simulink model "datarun_final"  (R2018a)
settings: Solver=VariableStepAuto  StartTime=0.0  StopTime=max(all_wheel_out_data(1,:))  RelTol=1e-3
PreLoadFcn:
  | load('all_wheel_out_data.mat');
  | load('bGbAtheta.mat');
  | load('pivot_offs_sws.mat');
  | load('ropod_kinmodel_pv.mat');
  | load('simple_bias_imu.mat');
  | load('simple_bias_gyro.mat');
values from neighbouring files (symbols this model uses):
  pivot_offs_sws = 1*[3.835 3.465 2.059 0.357]    [init_model.m]    (also in pivot_offs_sws.mat = [6.2589 0.5402 0.0584 0.0203])
  ropod_kinmodel_pv = [0.0525 0.0525 0.0525 0.0525 0.0525 0.0525 0.0525 0.0525 0.01 0.08 0.21 0.21 ... (18 elements, 1x18)]    [ropod_kinmodel_pv.mat]    (also in set_ropod_KinModparams.m = struct2array(ropod_kinmodel_param))
  simple_bias_gyro = [bias_gx; bias_gy; bias_gz]    [bias_simple.m]
  simple_bias_imu = [bias_x; bias_y]    [bias_simple.m]
undefined symbols (not defined in the file or in its folder): DiscIntNeverNeededParam
libraries: dspfdesign x12, simulink x5
settings Model: Creator=s151900  LastModifiedBy=s151900

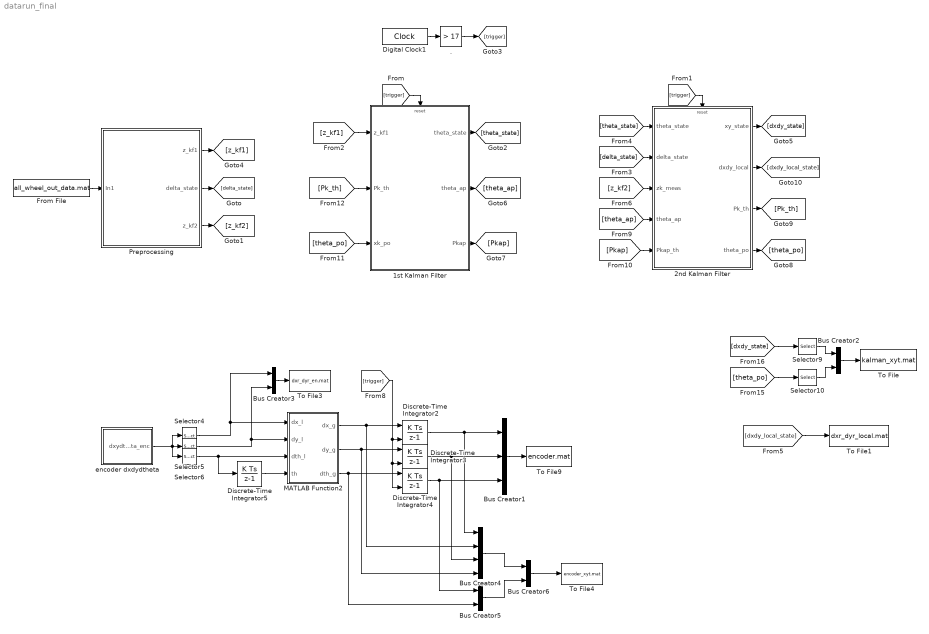
== system datarun_final ==
  . : simulink/Logic and Bit Operations/Compare To Constant  relop=>  const=17  OutDataTypeStr=boolean
  1st Kalman Filter : Subsystem  TreatAsAtomicUnit=on
  2nd Kalman Filter : Subsystem  TreatAsAtomicUnit=on
  Bus Creator1 : BusCreator  Inputs=3
  Bus Creator{2..3,5..6} (4 alike) : BusCreator  Inputs=2
  Bus Creator4 : BusCreator  Inputs=4
  Digital Clock1 : DigitalClock  SampleTime=0.001
  Discrete-Time Integrator2 : DiscreteIntegrator  gainval=1  ExternalReset=rising  SampleTime=-1  ICPrevOutput=DiscIntNeverNeededParam  ICPrevScaledInput=DiscIntNeverNeededParam
  Discrete-Time Integrator3 : DiscreteIntegrator  gainval=1  ExternalReset=rising  SampleTime=-1  ICPrevOutput=DiscIntNeverNeededParam  ICPrevScaledInput=DiscIntNeverNeededParam
  Discrete-Time Integrator4 : DiscreteIntegrator  gainval=1  ExternalReset=rising  InitialCondition=deg2rad(10)  SampleTime=-1  ICPrevOutput=DiscIntNeverNeededParam  ICPrevScaledInput=DiscIntNeverNeededParam
  Discrete-Time Integrator5 : DiscreteIntegrator  gainval=1  InitialCondition=deg2rad(10)  SampleTime=-1  ICPrevOutput=DiscIntNeverNeededParam  ICPrevScaledInput=DiscIntNeverNeededParam
  From File : FromFile  FileName=all_wheel_out_data.mat  SampleTime=0.001
  MATLAB Function2 : MATLAB Function  TreatAsAtomicUnit=on
  Preprocessing : Subsystem
  Selector10 : Selector  InputPortWidth=3  IndexOptions=Index vector (dialog)  Indices=[1 2]  OutputSizes=1
  Selector4 : Selector  InputPortWidth=3  IndexOptions=Index vector (dialog)  Indices=1  OutputSizes=1
  Selector5 : Selector  InputPortWidth=3  IndexOptions=Index vector (dialog)  Indices=2  OutputSizes=1
  Selector6 : Selector  InputPortWidth=3  IndexOptions=Index vector (dialog)  Indices=3  OutputSizes=1
  Selector9 : Selector  InputPortWidth=6  IndexOptions=Index vector (dialog)  Indices=[1 2 4 5]  OutputSizes=1
  To File : ToFile  Filename=kalman_xyt.mat  MatrixName=kalman_xyt
  To File1 : ToFile  Filename=dxr_dyr_local.mat  MatrixName=dxr_dyr_local
  To File3 : ToFile  Filename=dxr_dyr_en.mat  MatrixName=dxr_dyr_en
  To File4 : ToFile  Filename=encoder_xyt.mat  MatrixName=encoder_xyt
  To File9 : ToFile  Filename=encoder.mat
  encoder dxdydtheta : Subsystem
  wires:
  Digital Clock1/1 -> ./1
  From File/1 -> Preprocessing/1(In1)
  1st Kalman Filter/1(theta_state) -> [theta_state]
  Preprocessing/2(delta_state) -> [delta_state]
  Preprocessing/3(z_kf2) -> [z_kf2]
  [theta_state] -> 2nd Kalman Filter/1(theta_state)
  [delta_state] -> 2nd Kalman Filter/2(delta_state)
  [z_kf2] -> 2nd Kalman Filter/3(zk_meas)
  ./1 -> [trigger]
  [trigger] -> 1st Kalman Filter/Reset
  [trigger] -> 2nd Kalman Filter/Reset
  Preprocessing/1(z_kf1) -> [z_kf1]
  [z_kf1] -> 1st Kalman Filter/1(z_kf1)
  2nd Kalman Filter/1(xy_state) -> [dxdy_state]
  Bus Creator1/1 -> To File9/1
  Discrete-Time Integrator2/1 -> Bus Creator4/1, Bus Creator1/1
  Discrete-Time Integrator3/1 -> Bus Creator4/3, Bus Creator1/2
  Discrete-Time Integrator4/1 -> Bus Creator5/1, Bus Creator1/3
  1st Kalman Filter/2(theta_ap) -> [theta_ap]
  1st Kalman Filter/3("Pkap ") -> [Pkap]
  [theta_ap] -> 2nd Kalman Filter/4(theta_ap)
  [Pkap] -> 2nd Kalman Filter/5(Pkap_th)
  [theta_po] -> 1st Kalman Filter/3(xk_po)
  2nd Kalman Filter/4(theta_po) -> [theta_po]
  2nd Kalman Filter/3(Pk_th) -> [Pk_th]
  [Pk_th] -> 1st Kalman Filter/2(Pk_th)
  [theta_po] -> Selector10/1
  Bus Creator2/1 -> To File/1
  [dxdy_state] -> Selector9/1
  Selector10/1 -> Bus Creator2/2
  Selector9/1 -> Bus Creator2/1
  2nd Kalman Filter/2(dxdy_local) -> [dxdy_local_state]
  [dxdy_local_state] -> To File1/1
  Selector6/1 -> Discrete-Time Integrator5/1, MATLAB Function2/3(dth_l)
  Selector5/1 -> Bus Creator3/2, MATLAB Function2/2(dy_l)
  Bus Creator4/1 -> Bus Creator6/1
  encoder dxdydtheta/1(dxydtheta_enc) -> Selector4/1, Selector6/1, Selector5/1
  Bus Creator5/1 -> Bus Creator6/2
  MATLAB Function2/1(dx_g) -> Bus Creator4/2, Discrete-Time Integrator2/1
  Bus Creator3/1 -> To File3/1
  Selector4/1 -> Bus Creator3/1, MATLAB Function2/1(dx_l)
  Bus Creator6/1 -> To File4/1
  Discrete-Time Integrator5/1 -> MATLAB Function2/4(th)
  MATLAB Function2/2(dy_g) -> Discrete-Time Integrator3/1, Bus Creator4/4
  [trigger] -> Discrete-Time Integrator2/2, Discrete-Time Integrator4/2, Discrete-Time Integrator3/2
  MATLAB Function2/3(dth_g) -> Discrete-Time Integrator4/1, Bus Creator5/2

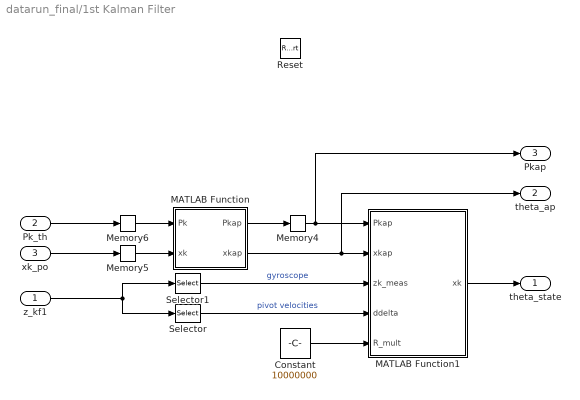
== system datarun_final/1st Kalman Filter ==
  z_kf1 : Inport  SampleTime=0.001
  Pk_th : Inport  Port=2
  xk_po : Inport  Port=3
  Reset : ResetPort  DisableCoverage=on
  Constant : Constant  Value=10000000
  MATLAB Function : MATLAB Function  TreatAsAtomicUnit=on
  MATLAB Function1 : MATLAB Function  TreatAsAtomicUnit=on
  Memory4 : Memory  InitialCondition=[1 0 0; 0 1 0; 0 0 1]  InheritSampleTime=on
  Memory5 : Memory  InitialCondition=[0;0;0]  InheritSampleTime=on
  Memory6 : Memory  InitialCondition=[1 0 0; 0 1 0; 0 0 1]  InheritSampleTime=on
  Selector : Selector  InputPortWidth=8  IndexOptions=Index vector (dialog)  Indices=[1 3 5 7]  OutputSizes=1
  Selector1 : Selector  InputPortWidth=8  IndexOptions=Index vector (dialog)  Indices=[2 4 6 8]  OutputSizes=1
  theta_state : Outport
  theta_ap : Outport  Port=2
  "Pkap " : Outport  Port=3
  wires:
  MATLAB Function/1(Pkap) -> Memory4/1
  Memory4/1 -> "Pkap "/1, MATLAB Function1/1(Pkap)
  MATLAB Function/2(xkap) -> theta_ap/1, MATLAB Function1/2(xkap)
  Memory6/1 -> MATLAB Function/1(Pk)
  Selector/1 -> MATLAB Function1/4(ddelta)  "pivot velocities"
  Selector1/1 -> MATLAB Function1/3(zk_meas)  "gyroscope"
  z_kf1/1 -> Selector1/1, Selector/1
  Constant/1 -> MATLAB Function1/5(R_mult)
  xk_po/1 -> Memory5/1
  MATLAB Function1/1(xk) -> theta_state/1
  Pk_th/1 -> Memory6/1
  Memory5/1 -> MATLAB Function/2(xk)

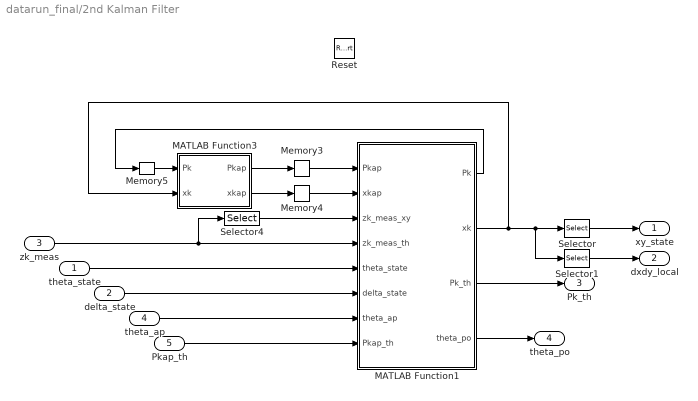
== system datarun_final/2nd Kalman Filter ==
  theta_state : Inport
  delta_state : Inport  Port=2
  zk_meas : Inport  Port=3
  theta_ap : Inport  Port=4
  Pkap_th : Inport  Port=5
  Reset : ResetPort  DisableCoverage=on
  MATLAB Function1 : MATLAB Function  TreatAsAtomicUnit=on
  MATLAB Function3 : MATLAB Function  TreatAsAtomicUnit=on
  Memory3 : Memory  InitialCondition=eye(10)  InheritSampleTime=on
  Memory4 : Memory  InitialCondition=zeros(10,1)  InheritSampleTime=on
  Memory5 : Memory  InitialCondition=eye(10)  InheritSampleTime=on
  Selector : Selector  InputPortWidth=10  IndexOptions=Index vector (dialog)  Indices=[1 2 3 4 5 6]  OutputSizes=1
  Selector1 : Selector  InputPortWidth=10  IndexOptions=Index vector (dialog)  Indices=[7 8 9 10]  OutputSizes=1
  Selector4 : Selector  InputPortWidth=20  IndexOptions=Index vector (dialog)  Indices=[2 3 4 5 7 8 9 10 12 13 14 15 17 18 19 20]  OutputSizes=1
  xy_state : Outport
  dxdy_local : Outport  Port=2
  Pk_th : Outport  Port=3
  theta_po : Outport  Port=4
  wires:
  Memory4/1 -> MATLAB Function1/2(xkap)
  Memory3/1 -> MATLAB Function1/1(Pkap)
  Memory5/1 -> MATLAB Function3/1(Pk)
  MATLAB Function1/1(Pk) -> Memory5/1
  MATLAB Function3/2(xkap) -> Memory4/1
  MATLAB Function3/1(Pkap) -> Memory3/1
  theta_state/1 -> MATLAB Function1/5(theta_state)
  delta_state/1 -> MATLAB Function1/6(delta_state)
  MATLAB Function1/3(Pk_th) -> Pk_th/1
  MATLAB Function1/4(theta_po) -> theta_po/1
  theta_ap/1 -> MATLAB Function1/7(theta_ap)
  Pkap_th/1 -> MATLAB Function1/8(Pkap_th)
  Selector4/1 -> MATLAB Function1/3(zk_meas_xy)
  zk_meas/1 -> Selector4/1, MATLAB Function1/4(zk_meas_th)
  MATLAB Function1/2(xk) -> Selector1/1, Selector/1, MATLAB Function3/2(xk)
  Selector/1 -> xy_state/1
  Selector1/1 -> dxdy_local/1

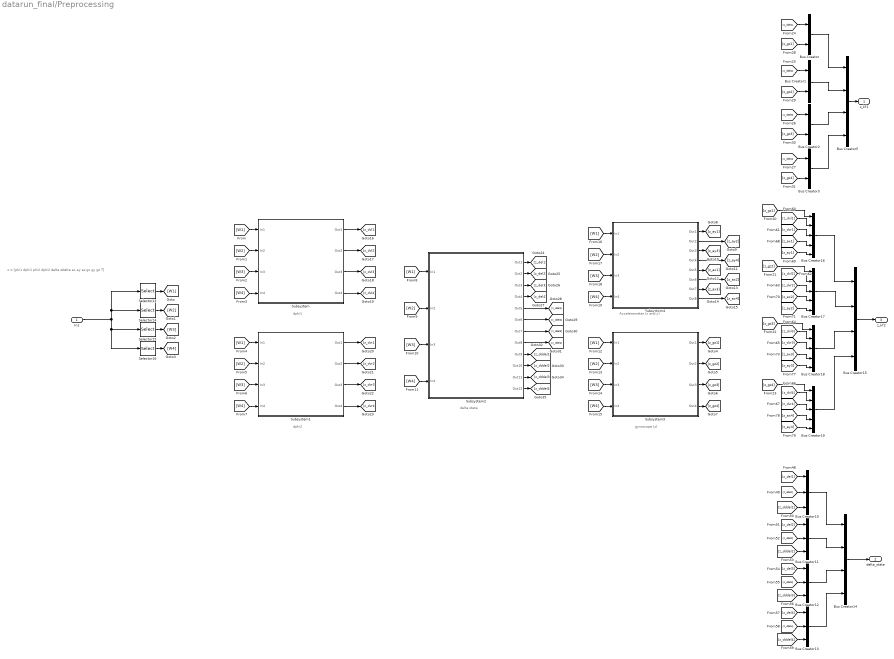
== system datarun_final/Preprocessing ==
  note: dphi1
  note: z = [phi1 dphi1 phi2 dphi2 delta ddelta ax ay az gx gy gz T]
  note: dphi2
  note: delta state
  note: gyroscope (z)
  note: Accelerometer (x and y)
  In1 : Inport
  Bus Creator{,1..3} (4 alike) : BusCreator  Inputs=2
  Bus Creator{10..13} (4 alike) : BusCreator  Inputs=3
  Bus Creator14 : BusCreator  Inputs=4
  Bus Creator15 : BusCreator  Inputs=4
  Bus Creator{16..19} (4 alike) : BusCreator  Inputs=5
  Bus Creator5 : BusCreator  Inputs=4
  Selector13 : Selector  InputPortWidth=160  IndexOptions=Index vector (dialog)  Indices=[5 6 17 18 29 30 33 34 35 36 37 38 39]  OutputSizes=1
  Selector14 : Selector  InputPortWidth=160  IndexOptions=Index vector (dialog)  Indices=[45 46 57 58 69 70 73 74 75 76 77 78 79]  OutputSizes=1
  Selector15 : Selector  InputPortWidth=160  IndexOptions=Index vector (dialog)  Indices=[85 86 97 98 109 110 113 114 115 116 117 118 119]  OutputSizes=1
  Selector16 : Selector  InputPortWidth=160  IndexOptions=Index vector (dialog)  Indices=[125 126 137 138 149 150 153 154 155 156 157 158 159]  OutputSizes=1
  Subsystem : Subsystem
  Subsystem1 : Subsystem
  Subsystem2 : Subsystem
  Subsystem3 : Subsystem
  Subsystem4 : Subsystem
  z_kf1 : Outport
  delta_state : Outport  Port=2
  z_kf2 : Outport  Port=3
  wires:
  Selector13/1 -> [W1]
  Selector16/1 -> [W4]
  In1/1 -> Selector15/1, Selector16/1, Selector14/1, Selector13/1
  Selector15/1 -> [W3]
  Selector14/1 -> [W2]
  [W1] -> Subsystem/1(In1)
  [W2] -> Subsystem/2(In2)
  [W3] -> Subsystem/3(In3)
  [W4] -> Subsystem/4(In4)
  [W1] -> Subsystem1/1(In1)
  [W2] -> Subsystem1/2(In2)
  [W4] -> Subsystem1/4(In4)
  [W3] -> Subsystem1/3(In3)
  [W4] -> Subsystem2/4(In4)
  [W3] -> Subsystem2/3(In3)
  [W2] -> Subsystem2/2(In2)
  [W1] -> Subsystem2/1(In1)
  [W4] -> Subsystem3/4(In4)
  [W3] -> Subsystem3/3(In3)
  [W2] -> Subsystem3/2(In2)
  [W1] -> Subsystem3/1(In1)
  [W4] -> Subsystem4/4(In4)
  [W3] -> Subsystem4/3(In3)
  [W2] -> Subsystem4/2(In2)
  [W1] -> Subsystem4/1(In1)
  Subsystem3/1(Out1) -> [z_gz1]
  Subsystem3/2(Out2) -> [z_gz2]
  Subsystem3/3(Out3) -> [z_gz3]
  Subsystem3/4(Out4) -> [z_gz4]
  Subsystem4/1(Out1) -> [z_ay1]
  Subsystem4/2(Out2) -> [z_ay2]
  Subsystem4/3(Out3) -> [z_ay3]
  Subsystem4/4(Out4) -> [z_ay4]
  Subsystem4/5(Out5) -> [z_ax1]
  Subsystem4/6(Out6) -> [z_ax2]
  Subsystem4/7(Out7) -> [z_ax3]
  Subsystem4/8(Out8) -> [z_ax4]
  Subsystem/1(Out1) -> [z_dvl1]
  Subsystem/2(Out2) -> [z_dvl2]
  Subsystem/3(Out3) -> [z_dvl3]
  Subsystem/4(Out4) -> [z_dvl4]
  Subsystem2/1(Out1) -> [z_del1]
  Subsystem2/2(Out2) -> [z_del2]
  Subsystem2/3(Out3) -> [z_del3]
  Subsystem2/4(Out4) -> [z_del4]
  Subsystem2/5(Out5) -> [z_ddel1]
  Subsystem2/6(Out6) -> [z_ddel2]
  Subsystem2/7(Out7) -> [z_ddel3]
  Subsystem2/8(Out8) -> [z_ddel4]
  Subsystem2/9(Out9) -> [z_dddel1]
  Subsystem2/10(Out10) -> [z_dddel2]
  Subsystem2/11(Out11) -> [z_dddel3]
  Subsystem2/12(Out12) -> [z_dddel4]
  [z_del2] -> Bus Creator11/1
  [z_dddel2] -> Bus Creator11/3
  [z_dddel3] -> Bus Creator12/3
  Bus Creator12/1 -> Bus Creator14/3
  [z_ddel1] -> Bus Creator10/2
  [z_ddel3] -> Bus Creator12/2
  [z_dddel4] -> Bus Creator13/3
  Bus Creator14/1 -> delta_state/1
  [z_del3] -> Bus Creator12/1
  Bus Creator10/1 -> Bus Creator14/1
  Bus Creator11/1 -> Bus Creator14/2
  [z_ddel4] -> Bus Creator13/2
  [z_del4] -> Bus Creator13/1
  Bus Creator13/1 -> Bus Creator14/4
  [z_ddel2] -> Bus Creator11/2
  [z_del1] -> Bus Creator10/1
  [z_dddel1] -> Bus Creator10/3
  Bus Creator19/1 -> Bus Creator15/4
  Bus Creator17/1 -> Bus Creator15/2
  Bus Creator15/1 -> z_kf2/1
  Bus Creator16/1 -> Bus Creator15/1
  Bus Creator18/1 -> Bus Creator15/3
  [z_dvr1] -> Bus Creator16/3
  [z_dvr2] -> Bus Creator17/3
  [z_dvl2] -> Bus Creator17/2
  [z_dvr3] -> Bus Creator18/3
  [z_dvl3] -> Bus Creator18/2
  [z_dvr4] -> Bus Creator19/3
  [z_dvl4] -> Bus Creator19/2
  [z_dvl1] -> Bus Creator16/2
  [z_ax1] -> Bus Creator16/4
  [z_ax2] -> Bus Creator17/4
  [z_ax3] -> Bus Creator18/4
  [z_ax4] -> Bus Creator19/4
  [z_ay1] -> Bus Creator16/5
  [z_ay2] -> Bus Creator17/5
  [z_ay3] -> Bus Creator18/5
  [z_ay4] -> Bus Creator19/5
  [z_gz4] -> Bus Creator3/2
  [z_gz3] -> Bus Creator2/2
  [z_ddel3] -> Bus Creator2/1
  [z_gz2] -> Bus Creator1/2
  [z_ddel4] -> Bus Creator3/1
  Bus Creator1/1 -> Bus Creator5/2
  [z_ddel1] -> Bus Creator/1
  Bus Creator2/1 -> Bus Creator5/3
  [z_gz1] -> Bus Creator/2
  Bus Creator3/1 -> Bus Creator5/4
  [z_ddel2] -> Bus Creator1/1
  Bus Creator/1 -> Bus Creator5/1
  Bus Creator5/1 -> z_kf1/1
  [z_gz1] -> Bus Creator16/1
  [z_gz2] -> Bus Creator17/1
  [z_gz3] -> Bus Creator18/1
  [z_gz4] -> Bus Creator19/1
  Subsystem1/1(Out1) -> [z_dvr1]
  Subsystem1/4(Out4) -> [z_dvr4]
  Subsystem1/3(Out3) -> [z_dvr3]
  Subsystem1/2(Out2) -> [z_dvr2]

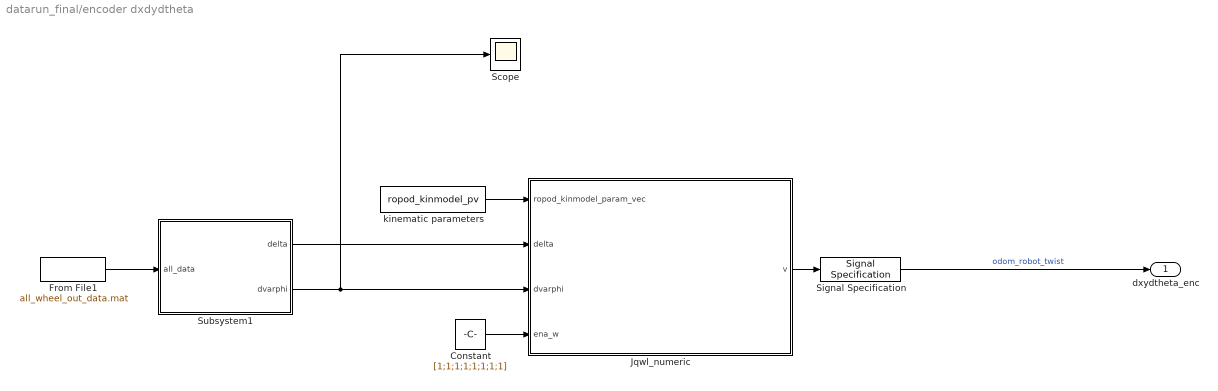
== system datarun_final/encoder dxdydtheta ==
  Constant : Constant  Value=[1;1;1;1;1;1;1;1]
  From File1 : FromFile  FileName=all_wheel_out_data.mat  SampleTime=0.001
  Jqwl_numeric : MATLAB Function  TreatAsAtomicUnit=on
  Scope : Scope
  Signal Specification : SignalSpecification  Dimensions=[3 1]
  Subsystem1 : Subsystem
  kinematic parameters : Constant  Value=ropod_kinmodel_pv
  dxydtheta_enc : Outport
  wires:
  Subsystem1/1(delta) -> Jqwl_numeric/2(delta)
  From File1/1 -> Subsystem1/1(all_data)
  kinematic parameters/1 -> Jqwl_numeric/1(ropod_kinmodel_param_vec)
  Constant/1 -> Jqwl_numeric/4(ena_w)
  Subsystem1/2(dvarphi) -> Scope/1, Jqwl_numeric/3(dvarphi)
  Jqwl_numeric/1(v) -> Signal Specification/1
  Signal Specification/1 -> dxydtheta_enc/1  "odom_robot_twist"

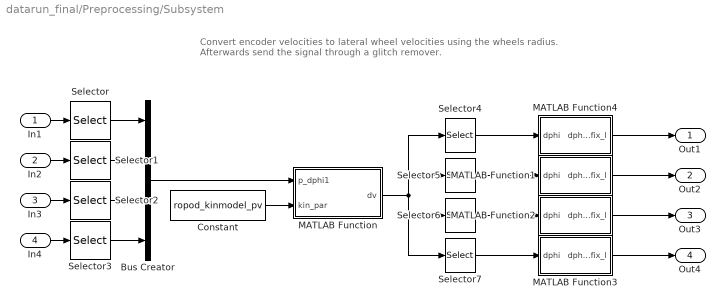
== system datarun_final/Preprocessing/Subsystem ==
  note: Convert encoder velocities to lateral wheel velocities using the wheels radius.
      | Afterwards send the signal through a glitch remover.
  In1 : Inport
  In2 : Inport  Port=2
  In3 : Inport  Port=3
  In4 : Inport  Port=4
  Bus Creator : BusCreator  Inputs=4
  Constant : Constant  Value=ropod_kinmodel_pv
  MATLAB Function : MATLAB Function  TreatAsAtomicUnit=on
  MATLAB Function1 : MATLAB Function  TreatAsAtomicUnit=on
  MATLAB Function2 : MATLAB Function  TreatAsAtomicUnit=on
  MATLAB Function3 : MATLAB Function  TreatAsAtomicUnit=on
  MATLAB Function4 : MATLAB Function  TreatAsAtomicUnit=on
  Selector{,1..3} (4 alike) : Selector  InputPortWidth=13  IndexOptions=Index vector (dialog)  Indices=2  OutputSizes=1
  Selector4 : Selector  InputPortWidth=4  IndexOptions=Index vector (dialog)  Indices=1  OutputSizes=1
  Selector5 : Selector  InputPortWidth=4  IndexOptions=Index vector (dialog)  Indices=2  OutputSizes=1
  Selector6 : Selector  InputPortWidth=4  IndexOptions=Index vector (dialog)  Indices=3  OutputSizes=1
  Selector7 : Selector  InputPortWidth=4  IndexOptions=Index vector (dialog)  Indices=4  OutputSizes=1
  Out1 : Outport
  Out2 : Outport  Port=2
  Out3 : Outport  Port=3
  Out4 : Outport  Port=4
  wires:
  In4/1 -> Selector3/1
  In2/1 -> Selector1/1
  In3/1 -> Selector2/1
  In1/1 -> Selector/1
  Selector1/1 -> Bus Creator/2
  Selector2/1 -> Bus Creator/3
  Selector3/1 -> Bus Creator/4
  Bus Creator/1 -> MATLAB Function/1(p_dphi1)
  Constant/1 -> MATLAB Function/2(kin_par)
  Selector7/1 -> MATLAB Function3/1(dphi)
  MATLAB Function/1(dv) -> Selector5/1, Selector4/1, Selector6/1, Selector7/1
  Selector4/1 -> MATLAB Function4/1(dphi)
  Selector5/1 -> MATLAB Function1/1(dphi)
  Selector6/1 -> MATLAB Function2/1(dphi)
  MATLAB Function3/1(dphi_fix_l) -> Out4/1
  MATLAB Function2/1(dphi_fix_l) -> Out3/1
  MATLAB Function1/1(dphi_fix_l) -> Out2/1
  MATLAB Function4/1(dphi_fix_l) -> Out1/1
  Selector/1 -> Bus Creator/1

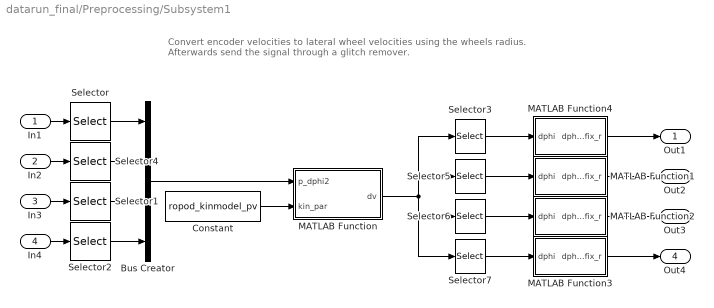
== system datarun_final/Preprocessing/Subsystem1 ==
  note: Convert encoder velocities to lateral wheel velocities using the wheels radius.
      | Afterwards send the signal through a glitch remover.
  In1 : Inport
  In2 : Inport  Port=2
  In3 : Inport  Port=3
  In4 : Inport  Port=4
  Bus Creator : BusCreator  Inputs=4
  Constant : Constant  Value=ropod_kinmodel_pv
  MATLAB Function : MATLAB Function  TreatAsAtomicUnit=on
  MATLAB Function1 : MATLAB Function  TreatAsAtomicUnit=on
  MATLAB Function2 : MATLAB Function  TreatAsAtomicUnit=on
  MATLAB Function3 : MATLAB Function  TreatAsAtomicUnit=on
  MATLAB Function4 : MATLAB Function  TreatAsAtomicUnit=on
  Selector{,1..2,4} (4 alike) : Selector  InputPortWidth=13  IndexOptions=Index vector (dialog)  Indices=4  OutputSizes=1
  Selector3 : Selector  InputPortWidth=4  IndexOptions=Index vector (dialog)  Indices=1  OutputSizes=1
  Selector5 : Selector  InputPortWidth=4  IndexOptions=Index vector (dialog)  Indices=2  OutputSizes=1
  Selector6 : Selector  InputPortWidth=4  IndexOptions=Index vector (dialog)  Indices=3  OutputSizes=1
  Selector7 : Selector  InputPortWidth=4  IndexOptions=Index vector (dialog)  Indices=4  OutputSizes=1
  Out1 : Outport
  Out2 : Outport  Port=2
  Out3 : Outport  Port=3
  Out4 : Outport  Port=4
  wires:
  In4/1 -> Selector2/1
  In2/1 -> Selector4/1
  In3/1 -> Selector1/1
  In1/1 -> Selector/1
  Constant/1 -> MATLAB Function/2(kin_par)
  Selector6/1 -> MATLAB Function2/1(dphi)
  Selector5/1 -> MATLAB Function1/1(dphi)
  Selector3/1 -> MATLAB Function4/1(dphi)
  Selector7/1 -> MATLAB Function3/1(dphi)
  MATLAB Function/1(dv) -> Selector5/1, Selector3/1, Selector6/1, Selector7/1
  Bus Creator/1 -> MATLAB Function/1(p_dphi2)
  Selector4/1 -> Bus Creator/2
  Selector/1 -> Bus Creator/1
  Selector1/1 -> Bus Creator/3
  Selector2/1 -> Bus Creator/4
  MATLAB Function4/1(dphi_fix_r) -> Out1/1
  MATLAB Function1/1(dphi_fix_r) -> Out2/1
  MATLAB Function2/1(dphi_fix_r) -> Out3/1
  MATLAB Function3/1(dphi_fix_r) -> Out4/1

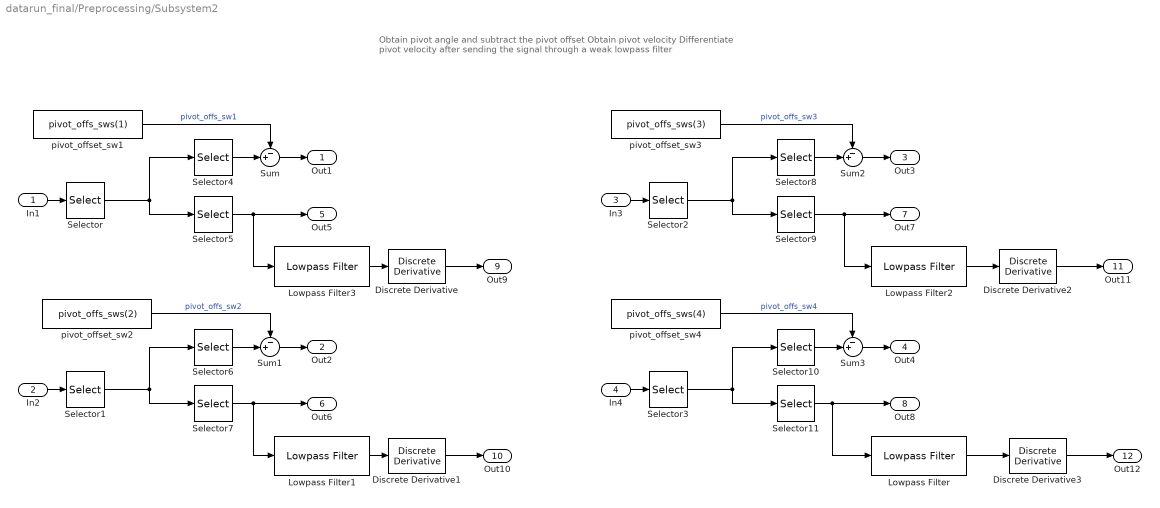
== system datarun_final/Preprocessing/Subsystem2 ==
  note: Obtain pivot angle and subtract the pivot offset
      | Obtain pivot velocity
      | Differentiate pivot velocity after sending the signal through a weak lowpass filter
  In1 : Inport
  In2 : Inport  Port=2
  In3 : Inport  Port=3
  In4 : Inport  Port=4
  Discrete Derivative{,1..3} (4 alike) : simulink/Discrete/Discrete Derivative  gainval=1  ICPrevScaledInput=0.0  OutMin=[]  OutMax=[]  OutDataType=fixdt(1, 16)  OutScaling=2^-10  DoSatur=off
  Lowpass Filter{,1..3} (4 alike) : dspfdesign/Lowpass Filter  FilterType=FIR  DesignForMinimumOrder=on  FilterOrder=50  PassbandFrequency=12  StopbandFrequency=50  PassbandRipple=0.1  StopbandAttenuation=80  InheritSampleRate=on  SampleRate=44100  SimulateUsing=Interpreted execution  roundingMode=Floor  coeffsDataTypeStr=fixdt(1,16)
  Selector{,1..3} (4 alike) : Selector  InputPortWidth=13  IndexOptions=Index vector (dialog)  Indices=[5 6]  OutputSizes=1
  Selector{4,6,8,10} (4 alike) : Selector  InputPortWidth=2  IndexOptions=Index vector (dialog)  Indices=1  OutputSizes=1
  Selector{5,7,9,11} (4 alike) : Selector  InputPortWidth=2  IndexOptions=Index vector (dialog)  Indices=2  OutputSizes=1
  Sum{,1..3} (4 alike) : Sum  Inputs=-+|
  pivot_offset_sw1 : Constant  Value=pivot_offs_sws(1)
  pivot_offset_sw2 : Constant  Value=pivot_offs_sws(2)
  pivot_offset_sw3 : Constant  Value=pivot_offs_sws(3)
  pivot_offset_sw4 : Constant  Value=pivot_offs_sws(4)
  Out1 : Outport
  Out2 : Outport  Port=2
  Out3 : Outport  Port=3
  Out4 : Outport  Port=4
  Out5 : Outport  Port=5
  Out6 : Outport  Port=6
  Out7 : Outport  Port=7
  Out8 : Outport  Port=8
  Out9 : Outport  Port=9
  Out10 : Outport  Port=10
  Out11 : Outport  Port=11
  Out12 : Outport  Port=12
  wires:
  In4/1 -> Selector3/1
  In2/1 -> Selector1/1
  In3/1 -> Selector2/1
  In1/1 -> Selector/1
  Selector5/1 -> Lowpass Filter3/1, Out5/1
  Selector/1 -> Selector5/1, Selector4/1
  Discrete Derivative/1 -> Out9/1
  Selector1/1 -> Selector7/1, Selector6/1
  Selector7/1 -> Lowpass Filter1/1, Out6/1
  Discrete Derivative1/1 -> Out10/1
  Selector9/1 -> Lowpass Filter2/1, Out7/1
  Selector2/1 -> Selector9/1, Selector8/1
  Selector11/1 -> Lowpass Filter/1, Out8/1
  Selector3/1 -> Selector11/1, Selector10/1
  Lowpass Filter/1 -> Discrete Derivative3/1
  Discrete Derivative3/1 -> Out12/1
  Discrete Derivative2/1 -> Out11/1
  Lowpass Filter3/1 -> Discrete Derivative/1
  Lowpass Filter1/1 -> Discrete Derivative1/1
  Lowpass Filter2/1 -> Discrete Derivative2/1
  pivot_offset_sw2/1 -> Sum1/1  "pivot_offs_sw2"
  pivot_offset_sw3/1 -> Sum2/1  "pivot_offs_sw3"
  pivot_offset_sw4/1 -> Sum3/1  "pivot_offs_sw4"
  pivot_offset_sw1/1 -> Sum/1  "pivot_offs_sw1"
  Selector4/1 -> Sum/2
  Sum/1 -> Out1/1
  Sum1/1 -> Out2/1
  Selector6/1 -> Sum1/2
  Selector8/1 -> Sum2/2
  Sum2/1 -> Out3/1
  Selector10/1 -> Sum3/2
  Sum3/1 -> Out4/1

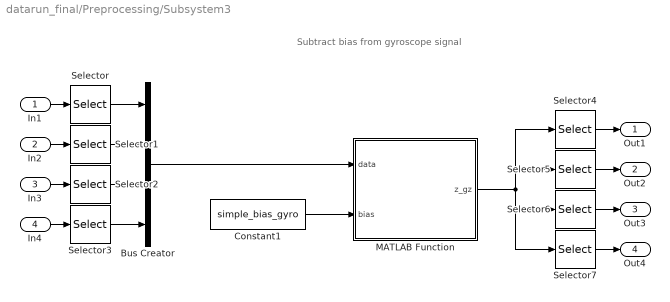
== system datarun_final/Preprocessing/Subsystem3 ==
  note: Subtract bias from gyroscope signal
  In1 : Inport
  In2 : Inport  Port=2
  In3 : Inport  Port=3
  In4 : Inport  Port=4
  Bus Creator : BusCreator  Inputs=4
  Constant1 : Constant  Value=simple_bias_gyro
  MATLAB Function : MATLAB Function  TreatAsAtomicUnit=on
  Selector{,1..3} (4 alike) : Selector  InputPortWidth=13  IndexOptions=Index vector (dialog)  Indices=[10 11 12]  OutputSizes=1
  Selector4 : Selector  InputPortWidth=4  IndexOptions=Index vector (dialog)  Indices=1  OutputSizes=1
  Selector5 : Selector  InputPortWidth=4  IndexOptions=Index vector (dialog)  Indices=2  OutputSizes=1
  Selector6 : Selector  InputPortWidth=4  IndexOptions=Index vector (dialog)  Indices=3  OutputSizes=1
  Selector7 : Selector  InputPortWidth=4  IndexOptions=Index vector (dialog)  Indices=4  OutputSizes=1
  Out1 : Outport
  Out2 : Outport  Port=2
  Out3 : Outport  Port=3
  Out4 : Outport  Port=4
  wires:
  In4/1 -> Selector3/1
  In2/1 -> Selector1/1
  In3/1 -> Selector2/1
  In1/1 -> Selector/1
  Constant1/1 -> MATLAB Function/2(bias)
  Selector/1 -> Bus Creator/1
  Selector1/1 -> Bus Creator/2
  Selector2/1 -> Bus Creator/3
  Selector3/1 -> Bus Creator/4
  Bus Creator/1 -> MATLAB Function/1(data)
  Selector4/1 -> Out1/1
  Selector5/1 -> Out2/1
  Selector6/1 -> Out3/1
  Selector7/1 -> Out4/1
  MATLAB Function/1(z_gz) -> Selector7/1, Selector6/1, Selector5/1, Selector4/1

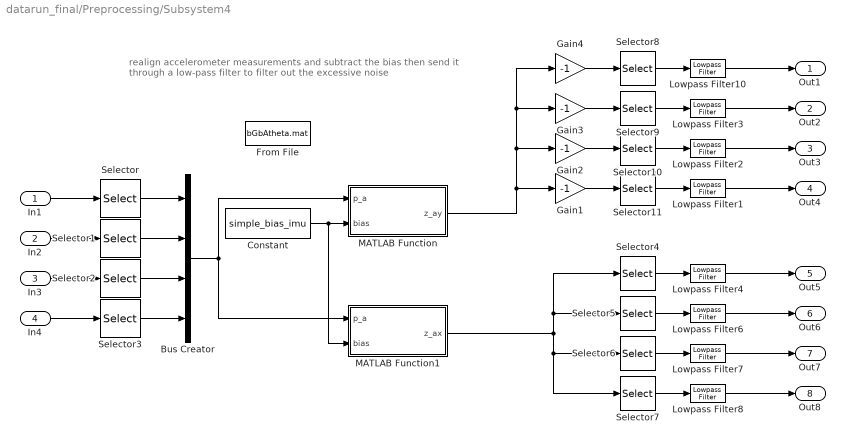
== system datarun_final/Preprocessing/Subsystem4 ==
  note: realign accelerometer measurements and subtract the bias
      | then send it through a low-pass filter to filter out the excessive noise
  In1 : Inport
  In2 : Inport  Port=2
  In3 : Inport  Port=3
  In4 : Inport  Port=4
  Bus Creator : BusCreator  Inputs=4
  Constant : Constant  Value=simple_bias_imu
  From File : FromFile  FileName=bGbAtheta.mat  SampleTime=0
  Gain{1..4} (4 alike) : Gain  Gain=-1
  Lowpass Filter{1..3,6..8} (6 alike) : dspfdesign/Lowpass Filter  FilterType=IIR  DesignForMinimumOrder=on  FilterOrder=50  PassbandFrequency=20  StopbandFrequency=100  PassbandRipple=0.1  StopbandAttenuation=10  InheritSampleRate=on  SampleRate=1000  SimulateUsing=Interpreted execution  roundingMode=Floor  coeffsDataTypeStr=fixdt(1,16)
  Lowpass Filter10 : dspfdesign/Lowpass Filter  FilterType=IIR  DesignForMinimumOrder=on  FilterOrder=50  PassbandFrequency=20  StopbandFrequency=50  PassbandRipple=0.1  StopbandAttenuation=4  InheritSampleRate=off  SampleRate=1000  SimulateUsing=Interpreted execution  roundingMode=Floor  coeffsDataTypeStr=fixdt(1,16)
  Lowpass Filter4 : dspfdesign/Lowpass Filter  FilterType=IIR  DesignForMinimumOrder=on  FilterOrder=50  PassbandFrequency=20  StopbandFrequency=100  PassbandRipple=0.1  StopbandAttenuation=10  InheritSampleRate=off  SampleRate=1000  SimulateUsing=Interpreted execution  roundingMode=Floor  coeffsDataTypeStr=fixdt(1,16)
  MATLAB Function : MATLAB Function  TreatAsAtomicUnit=on
  MATLAB Function1 : MATLAB Function  TreatAsAtomicUnit=on
  Selector{,1..3} (4 alike) : Selector  InputPortWidth=13  IndexOptions=Index vector (dialog)  Indices=[7 8 9]  OutputSizes=1
  Selector10 : Selector  InputPortWidth=4  IndexOptions=Index vector (dialog)  Indices=3  OutputSizes=1
  Selector11 : Selector  InputPortWidth=4  IndexOptions=Index vector (dialog)  Indices=4  OutputSizes=1
  Selector4 : Selector  InputPortWidth=4  IndexOptions=Index vector (dialog)  Indices=1  OutputSizes=1
  Selector5 : Selector  InputPortWidth=4  IndexOptions=Index vector (dialog)  Indices=2  OutputSizes=1
  Selector6 : Selector  InputPortWidth=4  IndexOptions=Index vector (dialog)  Indices=3  OutputSizes=1
  Selector7 : Selector  InputPortWidth=4  IndexOptions=Index vector (dialog)  Indices=4  OutputSizes=1
  Selector8 : Selector  InputPortWidth=4  IndexOptions=Index vector (dialog)  Indices=1  OutputSizes=1
  Selector9 : Selector  InputPortWidth=4  IndexOptions=Index vector (dialog)  Indices=2  OutputSizes=1
  Out1 : Outport
  Out2 : Outport  Port=2
  Out3 : Outport  Port=3
  Out4 : Outport  Port=4
  Out5 : Outport  Port=5
  Out6 : Outport  Port=6
  Out7 : Outport  Port=7
  Out8 : Outport  Port=8
  wires:
  In4/1 -> Selector3/1
  In2/1 -> Selector1/1
  In3/1 -> Selector2/1
  In1/1 -> Selector/1
  Selector/1 -> Bus Creator/1
  Selector1/1 -> Bus Creator/2
  Selector2/1 -> Bus Creator/3
  Selector3/1 -> Bus Creator/4
  Bus Creator/1 -> MATLAB Function1/1(p_a), MATLAB Function/1(p_a)
  Selector4/1 -> Lowpass Filter4/1
  Selector5/1 -> Lowpass Filter6/1
  Selector6/1 -> Lowpass Filter7/1
  Selector7/1 -> Lowpass Filter8/1
  Selector8/1 -> Lowpass Filter10/1
  Selector9/1 -> Lowpass Filter3/1
  Selector10/1 -> Lowpass Filter2/1
  Selector11/1 -> Lowpass Filter1/1
  MATLAB Function/1(z_ay) -> Gain1/1, Gain2/1, Gain3/1, Gain4/1
  Gain1/1 -> Selector11/1
  Gain2/1 -> Selector10/1
  Gain3/1 -> Selector9/1
  Gain4/1 -> Selector8/1
  Lowpass Filter10/1 -> Out1/1
  Lowpass Filter3/1 -> Out2/1
  Lowpass Filter2/1 -> Out3/1
  Lowpass Filter1/1 -> Out4/1
  MATLAB Function1/1(z_ax) -> Selector6/1, Selector7/1, Selector5/1, Selector4/1
  Lowpass Filter4/1 -> Out5/1
  Lowpass Filter6/1 -> Out6/1
  Lowpass Filter7/1 -> Out7/1
  Lowpass Filter8/1 -> Out8/1
  Constant/1 -> MATLAB Function1/2(bias), MATLAB Function/2(bias)

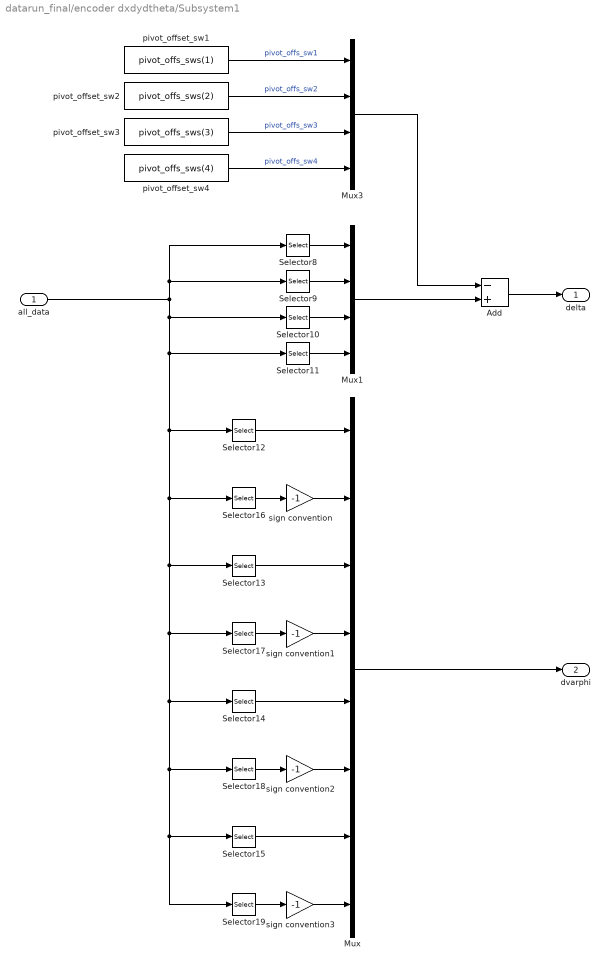
== system datarun_final/encoder dxdydtheta/Subsystem1 ==
  all_data : Inport
  Add : Sum  Inputs=-+
  Mux : Mux  Inputs=8
  Mux1 : Mux
  Mux3 : Mux
  Selector10 : Selector  InputPortWidth=160  IndexOptions=Index vector (dialog)  Indices=109  OutputSizes=1
  Selector11 : Selector  InputPortWidth=160  IndexOptions=Index vector (dialog)  Indices=149  OutputSizes=1
  Selector12 : Selector  InputPortWidth=160  IndexOptions=Index vector (dialog)  Indices=6  OutputSizes=1
  Selector13 : Selector  InputPortWidth=160  IndexOptions=Index vector (dialog)  Indices=46  OutputSizes=1
  Selector14 : Selector  InputPortWidth=160  IndexOptions=Index vector (dialog)  Indices=86  OutputSizes=1
  Selector15 : Selector  InputPortWidth=160  IndexOptions=Index vector (dialog)  Indices=126  OutputSizes=1
  Selector16 : Selector  InputPortWidth=160  IndexOptions=Index vector (dialog)  Indices=18  OutputSizes=1
  Selector17 : Selector  InputPortWidth=160  IndexOptions=Index vector (dialog)  Indices=58  OutputSizes=1
  Selector18 : Selector  InputPortWidth=160  IndexOptions=Index vector (dialog)  Indices=98  OutputSizes=1
  Selector19 : Selector  InputPortWidth=160  IndexOptions=Index vector (dialog)  Indices=138  OutputSizes=1
  Selector8 : Selector  InputPortWidth=160  IndexOptions=Index vector (dialog)  Indices=29  OutputSizes=1
  Selector9 : Selector  InputPortWidth=160  IndexOptions=Index vector (dialog)  Indices=69  OutputSizes=1
  pivot_offset_sw1 : Constant  Value=pivot_offs_sws(1)
  pivot_offset_sw2 : Constant  Value=pivot_offs_sws(2)
  pivot_offset_sw3 : Constant  Value=pivot_offs_sws(3)
  pivot_offset_sw4 : Constant  Value=pivot_offs_sws(4)
  sign convention{,1..3} (4 alike) : Gain  Gain=-1
  delta : Outport
  dvarphi : Outport  Port=2
  wires:
  Selector16/1 -> sign convention/1
  Selector17/1 -> sign convention1/1
  sign convention2/1 -> Mux/6
  sign convention/1 -> Mux/2
  Selector15/1 -> Mux/7
  Selector10/1 -> Mux1/3
  Selector11/1 -> Mux1/4
  Add/1 -> delta/1
  Mux3/1 -> Add/1
  Selector9/1 -> Mux1/2
  Selector8/1 -> Mux1/1
  all_data/1 -> Selector10/1, Selector19/1, Selector15/1, Selector18/1, Selector14/1, Selector17/1, Selector13/1, Selector16/1, Selector12/1, Selector11/1, Selector9/1, Selector8/1
  Mux1/1 -> Add/2
  sign convention3/1 -> Mux/8
  Selector12/1 -> Mux/1
  Mux/1 -> dvarphi/1
  Selector13/1 -> Mux/3
  sign convention1/1 -> Mux/4
  Selector14/1 -> Mux/5
  Selector18/1 -> sign convention2/1
  Selector19/1 -> sign convention3/1
  pivot_offset_sw3/1 -> Mux3/3  "pivot_offs_sw3"
  pivot_offset_sw1/1 -> Mux3/1  "pivot_offs_sw1"
  pivot_offset_sw4/1 -> Mux3/4  "pivot_offs_sw4"
  pivot_offset_sw2/1 -> Mux3/2  "pivot_offs_sw2"

== matlab function datarun_final/2nd Kalman Filter/MATLAB Function1 ==
  data: Pkap input; Pk output; xkap input; zk_meas_xy input; zk_meas_th input; theta_state input; delta_state input; xk output; theta_ap input; Pkap_th input; Pk_th output; theta_po output
%% Second Kalman filter (location) update stage
% J.P.M. Verhagen
% BEP: Odometry and localization esitmation of a mobile robot with multiple
% swivel wheels
% Commented on: 27-01-2019
function [Pk, xk,Pk_th,theta_po] = fcn(Pkap, xkap, zk_meas_xy, zk_meas_th, theta_state, delta_state,theta_ap,Pkap_th)
%% Stating constants
xr = [0.21 -0.21  0.21 -0.21]; % distance of pivots from center of robot
yr = [0.21  0.21 -0.21 -0.21];

delta   = [delta_state(1); delta_state(4); delta_state(7); delta_state(10)];
ddelta  = [delta_state(2); delta_state(5); delta_state(8); delta_state(11)];
dddelta = [delta_state(3); delta_state(6); delta_state(9); delta_state(12)];

theta   = theta_state(1);
dtheta  = theta_state(2);
ddtheta = theta_state(3);

dx   = xkap(2);
ddx  = xkap(3);
dy   = xkap(5);
ddy  = xkap(6);
dxr  = xkap(7);
ddxr = xkap(8);
dyr  = xkap(9);
ddyr = xkap(10);

sw = 0.01;          % offset pivot point and wheel axis
dw = 0.08;          % distance between wheels on a pivot
six = sw + 0.068;   % offset pivot point and IMU

%% Stating measurement predictions
wl_est = zeros(4,1);
wr_est = zeros(4,1);
ax_est = zeros(4,1);
ay_est = zeros(4,1);
wl_est_l = zeros(4,1);
wr_est_l = zeros(4,1);
ax_est_l = zeros(4,1);
ay_est_l = zeros(4,1);

for i = 1:4
    wl_est(i) = - (ddelta(i)*dw)/2 - (dtheta*dw)/2 + dx*cos(delta(i) + theta) + dy*sin(delta(i) + theta) - dtheta*yr(i)*cos(delta(i)) + dtheta*xr(i)*sin(delta(i));
    wr_est(i) =   (ddelta(i)*dw)/2 + (dtheta*dw)/2 + dx*cos(delta(i) + theta) + dy*sin(delta(i) + theta) - dtheta*yr(i)*cos(delta(i)) + dtheta*xr(i)*sin(delta(i));
    ax_est(i) = ddx*cos(delta(i) + theta) + ddy*sin(delta(i) + theta) + ddelta(i)^2*six + dtheta^2*six - ddtheta*yr(i)*cos(delta(i)) + ddtheta*xr(i)*sin(delta(i)) - dtheta^2*xr(i)*cos(delta(i)) - dtheta^2*yr(i)*sin(delta(i)) + 2*ddelta(i)*dtheta*six;
    ay_est(i) = ddy*cos(delta(i) + theta) - ddtheta*six - dddelta(i)*six - ddx*sin(delta(i) + theta) + ddtheta*xr(i)*cos(delta(i)) + ddtheta*yr(i)*sin(delta(i)) - dtheta^2*yr(i)*cos(delta(i)) + dtheta^2*xr(i)*sin(delta(i));

    wl_est_l(i) = - (ddelta(i)*dw)/2 - (dtheta*dw)/2 + dxr*cos(delta(i)) + dyr*sin(delta(i)) - dtheta*yr(i)*cos(delta(i)) + dtheta*xr(i)*sin(delta(i));
    wr_est_l(i) =   (ddelta(i)*dw)/2 + (dtheta*dw)/2 + dxr*cos(delta(i)) + dyr*sin(delta(i)) - dtheta*yr(i)*cos(delta(i)) + dtheta*xr(i)*sin(delta(i));
    ax_est_l(i) = ddxr*cos(delta(i)) + ddyr*sin(delta(i)) + ddelta(i)^2*six + dtheta^2*six - ddtheta*yr(i)*cos(delta(i)) + ddtheta*xr(i)*sin(delta(i)) - dtheta^2*xr(i)*cos(delta(i)) - dtheta^2*yr(i)*sin(delta(i)) + 2*ddelta(i)*dtheta*six;
    ay_est_l(i) = ddyr*cos(delta(i)) - ddtheta*six - dddelta(i)*six - ddxr*sin(delta(i)) + ddtheta*xr(i)*cos(delta(i)) + ddtheta*yr(i)*sin(delta(i)) - dtheta^2*yr(i)*cos(delta(i)) + dtheta^2*xr(i)*sin(delta(i));
end

%% Measurement mapping matrix
H = [0 cos(delta(1)+theta)  0 0 sin(delta(1)+theta) 0 0 0 0 0;
     0 cos(delta(1)+theta)  0 0 sin(delta(1)+theta) 0 0 0 0 0;
     0 0  cos(delta(1)+theta) 0 0 sin(delta(1)+theta) 0 0 0 0;
     0 0 -sin(delta(1)+theta) 0 0 cos(delta(1)+theta) 0 0 0 0;
     0 cos(delta(2)+theta) 0 0 sin(delta(2)+theta) 0  0 0 0 0;
     0 cos(delta(2)+theta) 0 0 sin(delta(2)+theta) 0  0 0 0 0;
     0 0  cos(delta(2)+theta) 0 0 sin(delta(2)+theta) 0 0 0 0;
     0 0 -sin(delta(2)+theta) 0 0 cos(delta(2)+theta) 0 0 0 0;
     0 cos(delta(3)+theta) 0 0 sin(delta(3)+theta) 0  0 0 0 0;
     0 cos(delta(3)+theta) 0 0 sin(delta(3)+theta) 0  0 0 0 0;
     0 0  cos(delta(3)+theta) 0 0 sin(delta(3)+theta) 0 0 0 0;
     0 0 -sin(delta(3)+theta) 0 0 cos(delta(3)+theta) 0 0 0 0;
     0 cos(delta(4)+theta) 0 0 sin(delta(4)+theta) 0  0 0 0 0;
     0 cos(delta(4)+theta) 0 0 sin(delta(4)+theta) 0  0 0 0 0;
     0 0  cos(delta(4)+theta) 0 0 sin(delta(4)+theta) 0 0 0 0;
     0 0 -sin(delta(4)+theta) 0 0 cos(delta(4)+theta) 0 0 0 0;
     
     0 0 0 0 0 0 cos(delta(1)) 0 sin(delta(1)) 0;
     0 0 0 0 0 0 cos(delta(1)) 0 sin(delta(1)) 0;
     0 0 0 0 0 0 0  cos(delta(1)) 0 sin(delta(1));
     0 0 0 0 0 0 0 -sin(delta(1)) 0 cos(delta(1));
     0 0 0 0 0 0 cos(delta(2)) 0 sin(delta(2)) 0;
     0 0 0 0 0 0 cos(delta(2)) 0 sin(delta(2)) 0;
     0 0 0 0 0 0 0  cos(delta(2)) 0 sin(delta(2));
     0 0 0 0 0 0 0 -sin(delta(2)) 0 cos(delta(2));
     0 0 0 0 0 0 cos(delta(3)) 0 sin(delta(3)) 0;
     0 0 0 0 0 0 cos(delta(3)) 0 sin(delta(3)) 0;
     0 0 0 0 0 0 0  cos(delta(3)) 0 sin(delta(3));
     0 0 0 0 0 0 0 -sin(delta(3)) 0 cos(delta(3));
     0 0 0 0 0 0 cos(delta(4)) 0 sin(delta(4)) 0;
     0 0 0 0 0 0 cos(delta(4)) 0 sin(delta(4)) 0;
     0 0 0 0 0 0 0  cos(delta(4)) 0 sin(delta(4));
     0 0 0 0 0 0 0 -sin(delta(4)) 0 cos(delta(4))];

zk_pred = [wl_est(1); wr_est(1); ax_est(1); ay_est(1);
           wl_est(2); wr_est(2); ax_est(2); ay_est(2);
           wl_est(3); wr_est(3); ax_est(3); ay_est(3);
           wl_est(4); wr_est(4); ax_est(4); ay_est(4);
           
           wl_est_l(1); wr_est_l(1); ax_est_l(1); ay_est_l(1);
           wl_est_l(2); wr_est_l(2); ax_est_l(2); ay_est_l(2);
           wl_est_l(3); wr_est_l(3); ax_est_l(3); ay_est_l(3);
           wl_est_l(4); wr_est_l(4); ax_est_l(4); ay_est_l(4)];

%% Measurement covariance matrix
res_l = zeros(4,1);
res_r = zeros(4,1);
R_wl = zeros(4,1);
R_wr = zeros(4,1);
R_st = 0.1;
for i = 1:4
    res_l(i) = zk_meas_xy(1+(i-1)*4) - zk_pred(1+(i-1)*4);
    res_r(i) = zk_meas_xy(2+(i-1)*4) - zk_pred(2+(i-1)*4);
    R_wl(i) = R_st + 40/2*(res_l(i))^4;
    R_wr(i) = R_st + 40/2*(res_l(i))^4;
end

R_mult = 0.1;
R_ax = 20;
R_ay = 40;
R_dyn_res = diag([R_wl(1) R_wr(1) R_ax R_ay ...
                  R_wl(2) R_wr(2) R_ax R_ay ...
                  R_wl(3) R_wr(3) R_ax R_ay ...
                  R_wl(4) R_wr(4) R_ax R_ay ...
                  R_wl(1) R_wr(1) R_ax R_ay ...
                  R_wl(2) R_wr(2) R_ax R_ay ...
                  R_wl(3) R_wr(3) R_ax R_ay ...
                  R_wl(4) R_wr(4) R_ax R_ay])*R_mult;

%% Stating Kalman Filter equations for position
I = eye(10);
Kk = Pkap*H'/(H*Pkap*H' + R_dyn_res);
xk = xkap + Kk*([zk_meas_xy;zk_meas_xy] - zk_pred);
Pk = (I - Kk*H)*Pkap;

%% Stating Kalman Filter equations for second orientation
H_th = [0 1 0;
        0 -dw/2-yr(1)*cos(delta(1))+xr(1)*sin(delta(1)) 0;
        0 +dw/2-yr(1)*cos(delta(1))+xr(1)*sin(delta(1)) 0;
        0 0 -yr(1)*cos(delta(1))+xr(1)*sin(delta(1));
        0 0 -six+xr(1)*cos(delta(1))+yr(1)*sin(delta(1));
        0 1 0;
        0 -dw/2-yr(2)*cos(delta(2))+xr(2)*sin(delta(2)) 0;
        0 +dw/2-yr(2)*cos(delta(2))+xr(2)*sin(delta(2)) 0;
        0 0 -yr(2)*cos(delta(2))+xr(2)*sin(delta(2));
        0 0 -six+xr(2)*cos(delta(2))+yr(2)*sin(delta(2));
        0 1 0;
        0 -dw/2-yr(3)*cos(delta(3))+xr(3)*sin(delta(3)) 0;
        0 +dw/2-yr(3)*cos(delta(3))+xr(3)*sin(delta(3)) 0;
        0 0 -yr(3)*cos(delta(3))+xr(3)*sin(delta(3));
        0 0 -six+xr(3)*cos(delta(3))+yr(3)*sin(delta(3));
        0 1 0;
        0 -dw/2-yr(4)*cos(delta(4))+xr(4)*sin(delta(4)) 0;
        0 +dw/2-yr(4)*cos(delta(4))+xr(4)*sin(delta(4)) 0;
        0 0 -yr(4)*cos(delta(4))+xr(4)*sin(delta(4));
        0 0 -six+xr(4)*cos(delta(4))+yr(4)*sin(delta(4))];

R_gz = 0.1;
R_mult_th = 1000;
R_th = diag([R_gz R_wl(1) R_wr(1) R_ax R_ay ...
             R_gz R_wl(2) R_wr(2) R_ax R_ay ...
             R_gz R_wl(3) R_wr(3) R_ax R_ay ...
             R_gz R_wl(4) R_wr(4) R_ax R_ay])*R_mult_th;    

gz_est = zeros(4,1);
for i = 1:4
    gz_est(i) = 0.5*(ddelta(i) + theta_ap(2));
end

zk_pred_th = [gz_est(1); wl_est(1); wr_est(1); ax_est(1); ay_est(1);
              gz_est(2); wl_est(2); wr_est(2); ax_est(2); ay_est(2);
              gz_est(3); wl_est(3); wr_est(3); ax_est(3); ay_est(3);
              gz_est(4); wl_est(4); wr_est(4); ax_est(4); ay_est(4)];

I_th = eye(3);
Kk_th = Pkap_th*H_th'/(H_th*Pkap_th*H_th' + R_th);
theta_po = theta_ap + Kk_th*(zk_meas_th - zk_pred_th);
Pk_th = (I_th - Kk_th*H_th)*Pkap_th;

== matlab function datarun_final/encoder dxdydtheta/Jqwl_numeric ==
  data: ropod_kinmodel_param_vec input; v output; delta input; dvarphi input; ena_w input
function v = Jqwl_numeric_wrapper(ropod_kinmodel_param_vec,  delta, dvarphi, ena_w)

v = Jqwl_numeric_function(ropod_kinmodel_param_vec, delta, dvarphi, ena_w);

end

== matlab function datarun_final/2nd Kalman Filter/MATLAB Function3 ==
  data: Pk input; Pkap output; xk input; xkap output
%% Second Kalman filter (location) predict stage
% J.P.M. Verhagen
% BEP: Odometry and localization esitmation of a mobile robot with multiple
% swivel wheels
% Commented on: 27-01-2019
function [Pkap, xkap] = fcn(Pk,xk)
%% Constant acceleration state transistion model
% state consits of [x dx ddx y dy ddy dxr ddxr dyr ddyr]
Ts = 1/1000; 
A = [1  Ts Ts^2/2 0  0  0      0 0 0 0;
     0  1  Ts     0  0  0      0 0 0 0;
     0  0  1      0  0  0      0 0 0 0;
     0  0  0      1  Ts Ts^2/2 0 0 0 0;
     0  0  0      0  1  Ts     0 0 0 0;
     0  0  0      0  0  1      0 0 0 0;
     0  0  0      0  0  0      1 Ts 0 0;
     0  0  0      0  0  0      0  1 0 0;
     0  0  0      0  0  0      0  0 1 Ts;
     0  0  0      0  0  0      0  0 0 1];

%% Process covariance matrix
Q_mult = 0.01;
Q = [Ts^4/4 Ts^3/3  Ts^2/2 0        0       0       0 0 0 0;
     Ts^3/3 Ts^2/2  Ts     0        0       0       0 0 0 0;
     Ts^2/2 Ts      1      0        0       0       0 0 0 0;
     0      0       0      Ts^4/4   Ts^3/3  Ts^2/2  0 0 0 0;
     0      0       0      Ts^3/3   Ts^2/2  Ts      0 0 0 0;
     0      0       0      Ts^2/2   Ts      1       0 0 0 0;
     0  0  0               0  0  0                  Ts^2/2 Ts  0       0;
     0  0  0               0  0  0                  Ts     1   0       0;
     0  0  0               0  0  0                  0      0   Ts^2/2  Ts;
     0  0  0               0  0  0                  0      0   Ts      1]*Q_mult;
     
%% Kalman filter equations
Pkap = A*Pk*A' + Q;
xkap = A*xk;

== matlab function datarun_final/Preprocessing/Subsystem/MATLAB Function1 ==
  data: dphi input; dphi_fix_l output
function dphi_fix_l = glitch_removal(dphi)

persistent last
if isempty(last)
    last = dphi;
    dphi_fix_l = dphi;
else
    last = [dphi last];
    last = last(1:2);
    if abs(last(1)-last(2)) > 0.2
        dphi_fix_l = last(2);
        last = [last(2) last(2)];
    else
        dphi_fix_l = last(1);
    end
end

== matlab function datarun_final/Preprocessing/Subsystem/MATLAB Function2 ==
  data: dphi input; dphi_fix_l output
function dphi_fix_l = glitch_removal(dphi)

persistent last
if isempty(last)
    last = dphi;
    dphi_fix_l = dphi;
else
    last = [dphi last];
    last = last(1:2);
    if abs(last(1)-last(2)) > 0.2
        dphi_fix_l = last(2);
        last = [last(2) last(2)];
    else
        dphi_fix_l = last(1);
    end
end

== matlab function datarun_final/Preprocessing/Subsystem/MATLAB Function3 ==
  data: dphi input; dphi_fix_l output
function dphi_fix_l = glitch_removal(dphi)

persistent last
if isempty(last)
    last = dphi;
    dphi_fix_l = dphi;
else
    last = [dphi last];
    last = last(1:2);
    if abs(last(1)-last(2)) > 0.2
        dphi_fix_l = last(2);
        last = [last(2) last(2)];
    else
        dphi_fix_l = last(1);
    end
end

== matlab function datarun_final/Preprocessing/Subsystem/MATLAB Function4 ==
  data: dphi input; dphi_fix_l output
function dphi_fix_l = glitch_removal(dphi)

persistent last
if isempty(last)
    last = dphi;
    dphi_fix_l = dphi;
else
    last = [dphi last];
    last = last(1:2);
    if abs(last(1)-last(2)) > 0.2
        dphi_fix_l = last(2);
        last = [last(2) last(2)];
    else
        dphi_fix_l = last(1);
    end
end

== matlab function datarun_final/Preprocessing/Subsystem1/MATLAB Function4 ==
  data: dphi input; dphi_fix_r output
function dphi_fix_r = glitch_removal(dphi)

persistent last
if isempty(last)
    last = dphi;
    dphi_fix_r = dphi;
else
    last = [dphi last];
    last = last(1:2);
    if abs(last(1)-last(2)) > 0.2
        dphi_fix_r = last(2);
        last = [last(2) last(2)];
    else
        dphi_fix_r = last(1);
    end
end

== matlab function datarun_final/Preprocessing/Subsystem1/MATLAB Function1 ==
  data: dphi input; dphi_fix_r output
function dphi_fix_r = glitch_removal(dphi)

persistent last
if isempty(last)
    last = dphi;
    dphi_fix_r = dphi;
else
    last = [dphi last];
    last = last(1:2);
    if abs(last(1)-last(2)) > 0.2
        dphi_fix_r = last(2);
        last = [last(2) last(2)];
    else
        dphi_fix_r = last(1);
    end
end

== matlab function datarun_final/Preprocessing/Subsystem1/MATLAB Function2 ==
  data: dphi input; dphi_fix_r output
function dphi_fix_r = glitch_removal(dphi)

persistent last
if isempty(last)
    last = dphi;
    dphi_fix_r = dphi;
else
    last = [dphi last];
    last = last(1:2);
    if abs(last(1)-last(2)) > 0.2
        dphi_fix_r = last(2);
        last = [last(2) last(2)];
    else
        dphi_fix_r = last(1);
    end
end

== matlab function datarun_final/Preprocessing/Subsystem1/MATLAB Function3 ==
  data: dphi input; dphi_fix_r output
function dphi_fix_r = glitch_removal(dphi)

persistent last
if isempty(last)
    last = dphi;
    dphi_fix_r = dphi;
else
    last = [dphi last];
    last = last(1:2);
    if abs(last(1)-last(2)) > 0.2
        dphi_fix_r = last(2);
        last = [last(2) last(2)];
    else
        dphi_fix_r = last(1);
    end
end

== matlab function datarun_final/Preprocessing/Subsystem3/MATLAB Function ==
  data: data input; z_gz output; bias input
function z_gz = fcn(data,bias)

b_g_x = bias(1,:);
b_g_y = bias(2,:);
b_g_z = bias(3,:);

gz = zeros(4,1);

for i = 1:4
    p_gx = data(1+(i-1)*3,:)-b_g_x(i);
    p_gy = data(2+(i-1)*3,:)-b_g_y(i);
    p_gz = data(3+(i-1)*3,:)-b_g_z(i);
    
    gz(i,:) = p_gy;
end

z_gz = gz;

== matlab function datarun_final/Preprocessing/Subsystem4/MATLAB Function ==
  data: p_a input; z_ay output; bias input
function z_ay = realign_ay(p_a,bias)

%% If bias is simple
b_a_y = bias(2,:);

ay = zeros(4,1);

for i = 1:4
    ay(i,:) = p_a(1+(i-1)*3,:) - b_a_y(i);
end

z_ay = ay;

%% If bias is complex
% b_a_y = bias(2,:);
% theta = bias(7,:);
% ay = zeros(4,1);
% 
% for i = 1:4
%     ay(i,:) = p_a(1+(i-1)*3,:)*cos(theta(i)) - b_a_y(i);
% end
% 
% z_ay = ay;

== matlab function datarun_final/Preprocessing/Subsystem4/MATLAB Function1 ==
  data: p_a input; z_ax output; bias input
function z_ax = realign_ax(p_a,bias)

%% If bias is simple
b_a_x = bias(1,:);

ax = zeros(4,1);

for i = 1:4
    ax(i,:) = -p_a(3+(i-1)*3,:) - b_a_x(i);
end

z_ax = ax;

%% If bias is complex
% b_a_x = bias(1,:);
% theta = bias(7,:);
% ax = zeros(4,1);
% 
% for i = 1:4
%     ax(i,:) = -p_a(3+(i-1)*3,:)*cos(theta(i)) + b_a_x(i);
% end
% 
% z_ax = ax;

== matlab function datarun_final/Preprocessing/Subsystem/MATLAB Function ==
  data: p_dphi1 input; dv output; kin_par input
function dv = fcn(p_dphi1,kin_par)

dphi = zeros(4,1);

for i = 1:4
    dphi(i) = p_dphi1(i)*kin_par(1+(i-1)*2);
end

dv = dphi;

== matlab function datarun_final/Preprocessing/Subsystem1/MATLAB Function ==
  data: p_dphi2 input; dv output; kin_par input
function dv = fcn(p_dphi2,kin_par)

dphi = zeros(4,1);

for i = 1:4
    dphi(i) = -p_dphi2(i)*kin_par(1+(i-1)*2);
end

dv = dphi;

== matlab function datarun_final/MATLAB Function2 ==
  data: dx_l input; dx_g output; dy_l input; dth_l input; dy_g output; dth_g output; th input
%% Mapping of local odometry obtained by encoder mapping to global velocities
% J.P.M. Verhagen
% BEP: Odometry and localization esitmation of a mobile robot with multiple
% swivel wheels
% Commented on: 27-01-2019

function [dx_g, dy_g, dth_g]= fcn(dx_l, dy_l, dth_l, th)

dth_g = -dth_l;

dx_g = dx_l * cos(th) + dy_l * sin(th);
dy_g = dy_l * cos(th) + dx_l * sin(th);

== matlab function datarun_final/1st Kalman Filter/MATLAB Function ==
  data: Pk input; Pkap output; xk input; xkap output
%% First Kalman filter (orientation) predict stage
% J.P.M. Verhagen
% BEP: Odometry and localization esitmation of a mobile robot with multiple
% swivel wheels
% Commented on: 27-01-2019

function [Pkap,xkap] = fcn(Pk,xk)
%% A priori state estimate based on constant acceleration state transition
Ts = 1/1000;
A = [1  Ts Ts^2/2 ;
     0  1  Ts     ; 
     0  0  1      ];


%% Process covariance matrix
Qmult = 100;

Q = [Ts^4/4 Ts^3/2 Ts^2/2 ;
     Ts^3/3 Ts^2/2 Ts     ;
     Ts^2/2 Ts     1      ]*Qmult;

%% Kalman filter equations
Pkap = A*Pk*A' + Q;
xkap = A*xk;

== matlab function datarun_final/1st Kalman Filter/MATLAB Function1 ==
  data: Pkap input; xkap input; xk output; zk_meas input; ddelta input; R_mult input
%% First Kalman filter (orientation) update stage
% J.P.M. Verhagen
% BEP: Odometry and localization esitmation of a mobile robot with multiple
% swivel wheels
% Commented on: 27-01-2019

function xk  = fcn(Pkap, xkap, zk_meas, ddelta,R_mult)
%% Measurement covariance matrix (based on noise variance of the gyroscope static measurements
Rmult = R_mult;
R = [0.000896   0           0           0;
     0          0.000920    0           0;
     0          0           0.000960    0;
     0          0           0           0.000802]*Rmult;

%% Measurement mapping matrix
H = [0 1 0;
     0 1 0;
     0 1 0;
     0 1 0];
 
H_full = [0 1 0 1 0 0 0;
          0 1 0 0 1 0 0;
          0 1 0 0 0 1 0;
          0 1 0 0 0 0 1];
   
zk_pred = 0.5*H_full*[xkap; ddelta]; % predicted measurements had to be divided by two to obtain the true value. Reasons unknown but this provides actual measurement prediction

%% Kalman filter equations
Kk = Pkap*H'/(H*Pkap*H' + R);
xk = xkap + Kk*(zk_meas - zk_pred);
